simulink model "IncCondAlg"  (R2019a)
settings: Solver=VariableStepAuto  StartTime=0.0  StopTime=10.0  RelTol=1e-3
libraries: simulink x4
settings Model: Creator=joao-  LastModifiedBy=joao-

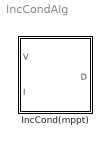
== system IncCondAlg ==
  IncCond(mppt) : Subsystem  mask{Value=0.001, InitialVCondition=20, InitialICondition=0, InitialDCondition=0.6, Period=0.001, PhaseDelay=1}
      mask prompts: Value "ΔD"; InitialVCondition "Vstart"; InitialICondition "Istart"; InitialDCondition "Dstart"; Period "Período(s)"; PhaseDelay "DelayInicial(s)"
      mask TypeOptions Value: dStep/Value
      mask TypeOptions InitialVCondition:
      | Triggered
      | Subsystem2/(k-1)1/InitialCondition
      mask TypeOptions InitialICondition:
      | Triggered
      | Subsystem1/(k-1)/InitialCondition
      mask TypeOptions InitialDCondition:
      | Triggered
      | Subsystem4/D(k-1)/InitialCondition
      mask TypeOptions Period: T (mppt)/Period
      mask TypeOptions PhaseDelay: T (mppt)/PhaseDelay
      mask Display: image('C:\Users\joao-\Desktop\mptt.png');

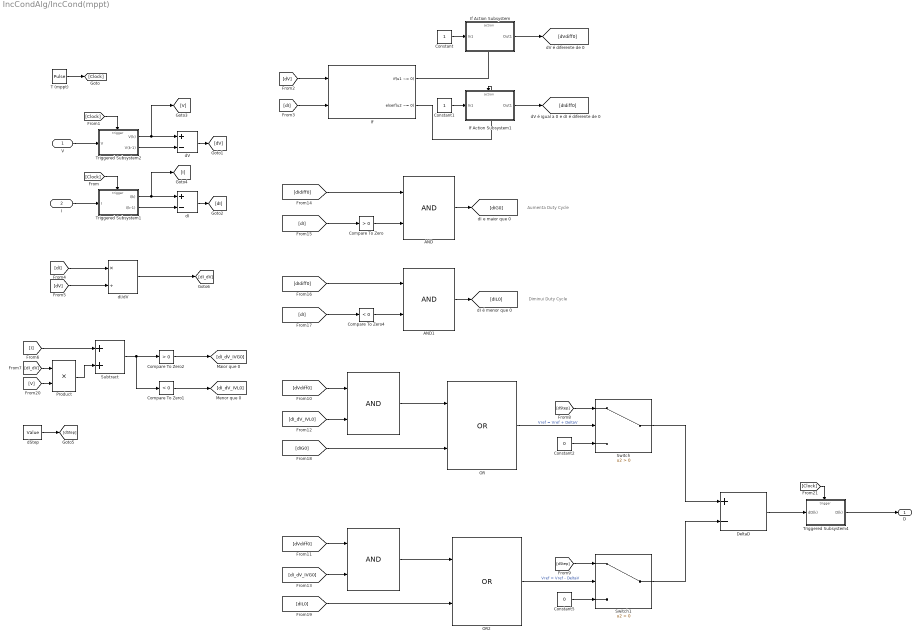
== system IncCondAlg/IncCond(mppt) ==
  note: Diminui Duty Cycle
  note: Aumenta Duty Cycle
  V : Inport
  I : Inport  Port=2
  " " : Logic  IconShape=distinctive  AllPortsSameDT=off  OutDataTypeStr=boolean
  " " : Logic  IconShape=distinctive  AllPortsSameDT=off  OutDataTypeStr=boolean
  " AND" : Logic  IconShape=distinctive  AllPortsSameDT=off  OutDataTypeStr=boolean
  " AND1" : Logic  IconShape=distinctive  AllPortsSameDT=off  OutDataTypeStr=boolean
  Compare To Zero : simulink/Logic and Bit Operations/Compare To Zero  relop=>  OutDataTypeStr=boolean
  Compare To Zero1 : simulink/Logic and Bit Operations/Compare To Zero  relop=<  OutDataTypeStr=boolean
  Compare To Zero2 : simulink/Logic and Bit Operations/Compare To Zero  relop=>  OutDataTypeStr=boolean
  Compare To Zero4 : simulink/Logic and Bit Operations/Compare To Zero  relop=<  OutDataTypeStr=boolean
  Constant : Constant
  Constant1 : Constant
  Constant2 : Constant  Value=0
  Constant5 : Constant  Value=0
  DeltaD : Sum  Inputs=+-
  If : If  NumInputs=2  IfExpression=u1 ~= 0  ElseIfExpressions=u2 ~= 0  ShowElse=off
  If Action Subsystem : Subsystem  TreatAsAtomicUnit=on
  If Action Subsystem1 : Subsystem  TreatAsAtomicUnit=on
  OR : Logic  Operator=OR  IconShape=distinctive  AllPortsSameDT=off  OutDataTypeStr=boolean
  OR2 : Logic  Operator=OR  IconShape=distinctive  AllPortsSameDT=off  OutDataTypeStr=boolean
  Product : Product
  Subtract : Sum
  Switch : Switch  Criteria=u2 > Threshold
  Switch1 : Switch  Criteria=u2 > Threshold
  T (mppt) : DiscretePulseGenerator  PulseType=Time based  Amplitude=5  Period=Period  PulseWidth=50  PhaseDelay=PhaseDelay
      settings: AttributesFormatString=%<Period>
  Triggered Subsystem1 : Subsystem  TreatAsAtomicUnit=on
  Triggered Subsystem2 : Subsystem  TreatAsAtomicUnit=on
  Triggered Subsystem4 : Subsystem  TreatAsAtomicUnit=on
  dI : Sum  Inputs=+-
  dI/dV : Product  Inputs=*/
  dStep : Constant  Value=Value
  dV : Sum  Inputs=+-
  "D " : Outport
  wires:
  I/1 -> Triggered Subsystem1/1(I)
  V/1 -> Triggered Subsystem2/1(V)
  T (mppt)/1 -> [Clock]
  [Clock] -> Triggered Subsystem2/Trigger
  [Clock] -> Triggered Subsystem1/Trigger
  Triggered Subsystem2/1(V(k)) -> dV/1, [V]
  Triggered Subsystem1/2(I(k-1)) -> dI/2
  Triggered Subsystem1/1(I(k)) -> [I], dI/1
  [dV] -> If/1
  [dI] -> If/2
  dI/1 -> [dI]
  [dV] -> dI/dV/2
  [I] -> Subtract/1
  [dI] -> dI/dV/1
  dI/dV/1 -> [dI_dV]
  Triggered Subsystem2/2(V(k-1)) -> dV/2
  dV/1 -> [dV]
  If/1 -> If Action Subsystem/Action
  If/2 -> If Action Subsystem1/Action
  [dI_dV_IVL0] -> " "/2
  [dVdiff0] -> " "/1
  [dVdiff0] -> " "/1
  [dI_dV_IVG0] -> " "/2
  " "/1 -> OR/1
  " "/1 -> OR2/1
  OR/1 -> Switch/2  "Vref = Vref + DeltaV"
  OR2/1 -> Switch1/2  "Vref = Vref - DeltaV"
  [dI] -> Compare To Zero/1
  [dIdiff0] -> " AND"/1
  Compare To Zero/1 -> " AND"/2
  Compare To Zero4/1 -> " AND1"/2
  [dIdiff0] -> " AND1"/1
  [dI] -> Compare To Zero4/1
  " AND"/1 -> [dIG0]
  " AND1"/1 -> [dIL0]
  [dIG0] -> OR/2
  [dIL0] -> OR2/2
  Constant/1 -> If Action Subsystem/1(In1)
  If Action Subsystem/1(Out1) -> [dVdiff0]
  Constant1/1 -> If Action Subsystem1/1(In1)
  If Action Subsystem1/1(Out1) -> [dIdiff0]
  Constant2/1 -> Switch/3
  [dStep] -> Switch/1
  [dStep] -> Switch1/1
  Constant5/1 -> Switch1/3
  Switch1/1 -> DeltaD/2
  Switch/1 -> DeltaD/1
  DeltaD/1 -> Triggered Subsystem4/1(dD(k))
  [Clock] -> Triggered Subsystem4/Trigger
  Triggered Subsystem4/1(D(k)) -> "D "/1
  [dI_dV] -> Product/1
  Product/1 -> Subtract/2
  [V] -> Product/2
  dStep/1 -> [dStep]
  Compare To Zero2/1 -> [dI_dV_IVG0]
  Subtract/1 -> Compare To Zero1/1, Compare To Zero2/1
  Compare To Zero1/1 -> [dI_dV_IVL0]

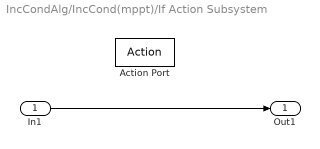
== system IncCondAlg/IncCond(mppt)/If Action Subsystem ==
  In1 : Inport
  Action Port : ActionPort
  Out1 : Outport
  wires:
  In1/1 -> Out1/1

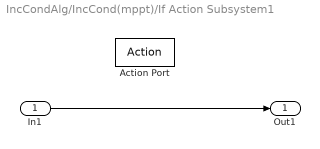
== system IncCondAlg/IncCond(mppt)/If Action Subsystem1 ==
  In1 : Inport
  Action Port : ActionPort
  Out1 : Outport
  wires:
  In1/1 -> Out1/1

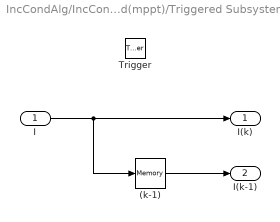
== system IncCondAlg/IncCond(mppt)/Triggered Subsystem1 ==
  I : Inport  LatchByDelayingOutsideSignal=on
  Trigger : TriggerPort  VariantControl=(inherit)
  (k-1) : Memory  InitialCondition=InitialICondition  InheritSampleTime=on  LinearizeMemory=on  LinearizeAsDelay=on
  I(k) : Outport
  I(k-1) : Outport  Port=2  InitialOutput=1
  wires:
  I/1 -> I(k)/1, (k-1)/1
  (k-1)/1 -> I(k-1)/1

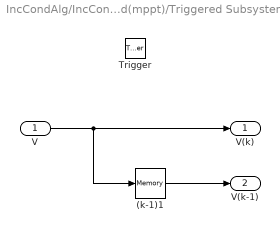
== system IncCondAlg/IncCond(mppt)/Triggered Subsystem2 ==
  V : Inport  LatchByDelayingOutsideSignal=on
  Trigger : TriggerPort  VariantControl=(inherit)
  (k-1)1 : Memory  InitialCondition=InitialVCondition  InheritSampleTime=on  LinearizeMemory=on  LinearizeAsDelay=on
  V(k) : Outport
  V(k-1) : Outport  Port=2  InitialOutput=20
  wires:
  (k-1)1/1 -> V(k-1)/1
  V/1 -> V(k)/1, (k-1)1/1

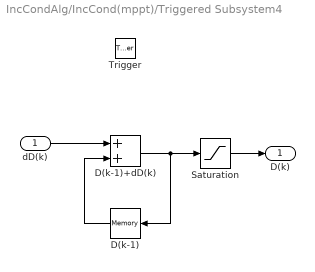
== system IncCondAlg/IncCond(mppt)/Triggered Subsystem4 ==
  dD(k) : Inport
  Trigger : TriggerPort  VariantControl=(inherit)
  D(k-1) : Memory  InitialCondition=InitialDCondition  InheritSampleTime=on  LinearizeMemory=on  LinearizeAsDelay=on
  D(k-1)+dD(k) : Sum
  Saturation : Saturate  UpperLimit=0.9  LowerLimit=0
  D(k) : Outport
  wires:
  dD(k)/1 -> D(k-1)+dD(k)/1
  D(k-1)/1 -> D(k-1)+dD(k)/2
  D(k-1)+dD(k)/1 -> Saturation/1, D(k-1)/1
  Saturation/1 -> D(k)/1
